simulink model "errore_offset_proporzionale"  (R2022b)
settings: Solver=VariableStepAuto  StartTime=0.0  StopTime=50  RelTol=1e-3
libraries: simulink x1
settings Model: Creator=giuli  LastModifiedBy=giuli

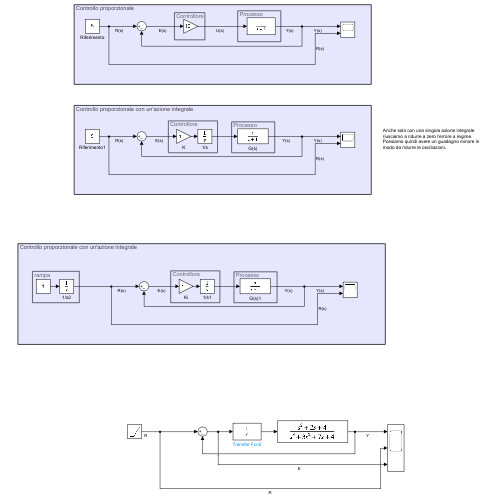
[thumbnail: Simulink's stored preview of the top-level diagram]
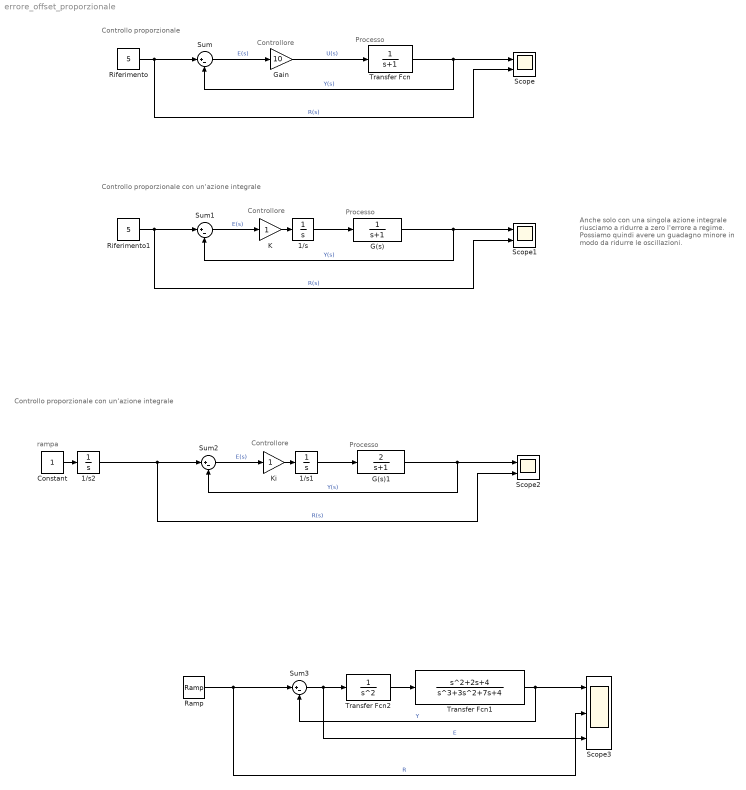
== system errore_offset_proporzionale ==
  note: rampa
  note: Anche solo con una singola azione integrale riusciamo a ridurre a zero l'errore a regime. Possiamo quindi avere un guadagno minore in modo da ridurre le oscillazioni.
  note: Processo
  note: Controllore
  note: Controllo proporzionale
  note: Controllo proporzionale con un'azione integrale
  note: Controllore
  note: Processo
  note: Controllore
  note: Controllo proporzionale con un'azione integrale
  note: Processo
  1/s : Integrator
  1/s1 : Integrator
  1/s2 : Integrator
  Constant : Constant
  G(s) : TransferFcn  Denominator=[1 1]
  G(s)1 : TransferFcn  Numerator=[2]  Denominator=[1 1]
  Gain : Gain  Gain=10
  K : Gain
  Ki : Gain
  Ramp : simulink/Sources/Ramp  slope=1  start=0  InitialOutput=0
  Riferimento : Constant  Value=5
  Riferimento1 : Constant  Value=5
  Scope : Scope  NumInputPorts=2
  Scope1 : Scope  NumInputPorts=2
  Scope2 : Scope  NumInputPorts=2
  Scope3 : Scope  NumInputPorts=3
  Sum{,1..3} (4 alike) : Sum  Inputs=|+-
  Transfer Fcn : TransferFcn  Denominator=[1 1]
  Transfer Fcn1 : TransferFcn  Numerator=[1 2 4]  Denominator=[1 3 7 4]
  Transfer Fcn2 : TransferFcn  Denominator=[1 0 0]
  wires:
  Gain/1 -> Transfer Fcn/1  "U(s)"
  Transfer Fcn/1 -> Sum/2, Scope/1  "Y(s)"
  Sum/1 -> Gain/1  "E(s)"
  Riferimento/1 -> Scope/2, Sum/1  "R(s)"
  Riferimento1/1 -> Scope1/2, Sum1/1  "R(s)"
  Sum1/1 -> K/1  "E(s)"
  G(s)/1 -> Sum1/2, Scope1/1  "Y(s)"
  K/1 -> 1/s/1
  1/s/1 -> G(s)/1
  1/s1/1 -> G(s)1/1
  1/s2/1 -> Scope2/2, Sum2/1  "R(s)"
  G(s)1/1 -> Sum2/2, Scope2/1  "Y(s)"
  Ki/1 -> 1/s1/1
  Sum2/1 -> Ki/1  "E(s)"
  Constant/1 -> 1/s2/1
  Transfer Fcn1/1 -> Sum3/2, Scope3/1  "Y"
  Ramp/1 -> Scope3/2, Sum3/1  "R"
  Sum3/1 -> Transfer Fcn2/1, Scope3/3  "E"
  Transfer Fcn2/1 -> Transfer Fcn1/1
